simulink model "E010_A1_ton_trunc_from_ideal_iqcot_20260628"  (R2024b)
settings: Solver=VariableStepAuto  StartTime=0.0  StopTime=0.54e-3  MaxStep=5e-9  RelTol=1e-3
undefined symbols (not defined in the file): A_init, A_lower, A_upper, Cout, DCR_L1, DCR_L2, DCR_L3, DCR_L4, E010_TonTrunc_Enable, ESR_C, IdealIQCOT_Enable, IL_adc_counts_per_A, IL_pk_limit_adc_neg, IL_pk_limit_adc_pos, Iload_final, Iload_initial, Iph, Iqcot_enable, kappa_cmd, Kiqcot, Kvc_iqcot, L, Lambda0_iqcot, Lambda_m2, rho_cmd, Ri_iqcot, t_load_step, Tblank, Tdead, Tiqcot_leak, Toff_min, Ton_cmd, Ton_iq_max, Ton_iq_min, Ts_ctrl, Tslot, Tss, Tton_trunc_min, Tton_trunc_window, Vc_bias_iqcot, Vcot_ramp_amp, Vcot_ramp_enable, Vhys, Vin, Vo_ref
libraries: simulink x29, spsCurrentMeasurementLib x8, spsMosfetLib x8, spsSeriesRLCBranchLib x5, spsVoltageMeasurementLib x5, spsDCVoltageSourceLib x4, spsControlledCurrentSourceLib x1, spsGroundLib x1, spspowerguiLib x1
(part 2 of 2)

== matlab function E010_A1_ton_trunc_from_ideal_iqcot_20260628/E010_TonTrunc3 ==
  data: ton_in input double size=1; ton_out output double size=1; t input double size=1; t_step input double size=1; t_window input double size=1; t_min input double size=1; enable input double size=1; trunc_active output double size=1
function [ton_out,trunc_active] = ton_trunc(ton_in,t,t_step,t_window,t_min,enable)
%#codegen
active = (enable > 0.5) && (t >= t_step) && (t <= (t_step + t_window));
trunc_active = double(active);
if active
    ton_out = min(ton_in, t_min);
else
    ton_out = ton_in;
end

== matlab function E010_A1_ton_trunc_from_ideal_iqcot_20260628/E010_TonTrunc4 ==
  data: ton_in input double size=1; ton_out output double size=1; t input double size=1; t_step input double size=1; t_window input double size=1; t_min input double size=1; enable input double size=1; trunc_active output double size=1
function [ton_out,trunc_active] = ton_trunc(ton_in,t,t_step,t_window,t_min,enable)
%#codegen
active = (enable > 0.5) && (t >= t_step) && (t <= (t_step + t_window));
trunc_active = double(active);
if active
    ton_out = min(ton_in, t_min);
else
    ton_out = ton_in;
end
